simulink model "early_return2_2018a"  (R2020a)
settings: Solver=VariableStepAuto  StartTime=0.0  StopTime=10.0  RelTol=1e-3
settings Model: Creator=apple  LastModifiedBy=apple

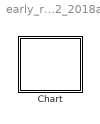
== system early_return2_2018a ==
  Chart : Stateflow chart  TreatAsAtomicUnit=on

== stateflow chart early_return2_2018a/Chart ==
  state A
    state A2
    state A1
    (default) -> A1
    A -> A1 : E
    A1 -> A2 : /{E}
  (default) -> A
  events: E local FUNCTION_CALL_EVENT
